simulink model "RobotX_ss_acousticsSKIP_dock_odoa_refer_model1021"  (R2014a)
settings: Solver=FixedStepDiscrete  StartTime=0.0  StopTime=inf  FixedStep=.25  RelTol=1e-3
undefined symbols (not defined in the file): Com1, Com2, Com3, Com4, DiscIntNeverNeededParam, standard
libraries: xpcseriallib x42, slrtlib x8, simulink x7, speedgoatlib x2, speedgoatlib_IO102 x1
(part 4 of 18)

== matlab function RobotX_ss_acousticsSKIP_dock_odoa_refer_model1021/Main FSM/ODOA/SLAM1/SLAM enabled/slammed ==
  data: mpa output; lm_data input; pre_part_positions input; part_positions output; positionboat input
%% SLAM by Chidananda Matada Shivananda
%  Copyright 2010 Randolph Voorhies

%  Edited 2014 Nick DiLeo - Modifications for unknown data association
%  and multiple measurements in a single timestep
    
%  Edited 2014 Chidananda Matada Shivananda - Simulink compatability, New
%  clustering technique added

%  This program is free software: you can redistribute it and/or modify
%  it under the terms of the GNU General Public License as published by
%  the Free Software Foundation, either version 3 of the License, or
%  (at your option) any later version.
%
%  This program is distributed in the hope that it will be useful,
%  but WITHOUT ANY WARRANTY; without even the implied warranty of
%  MERCHANTABILITY or FITNESS FOR A PARTICULAR PURPOSE.  See the
%  GNU General Public License for more details.
%
%  You should have received a copy of the GNU General Public License
%  along with this program.  If not, see <http://www.gnu.org/licenses/>.

function [mpa,part_positions]   = slammed(lm_data,pre_part_positions,positionboat)

%% General comments

% the angles in radians
% the ditance in m

%% Initialisations.

persistent particles avg_robot;
num_particles = 50;

% the limits
max_read_distance = 10;
min_read_distance = 5;
min_read_angle = -67.5*pi/180; %radians- maximum read angle
max_read_angle = 67.5*pi/180;

% The initial starting position of the robot Use UTM coordinates from GPS
avg_robot_position = [0;0;0];% x y rotation

% The Gaussian variance of the movement commands
% Approximating there are only two drives
% movement_variance = [.1;.1];   % Left drive Right_drive
% M = [movement_variance(1), 0.0;
%      0.0, movement_variance(2)];
measurement_variance = [0.01; 0.01];   % Distance Angle
R = [measurement_variance(1), 0.0;
    0.0, measurement_variance(2)];

default_importance=0.001;

if isempty(particles)
    %  Particles
    %             w[1]
    %             position[1,3]
    %             num_landmarks[300] this is to keep history
    
    %             lm_weight[2,15]based on number of landmarks
    %             landmarks[15]
    %                         position[2,1]
    %                         E[2,2]
    %                         counter[1]
    particles=repmat(struct('w',1.0/num_particles,'position',avg_robot_position,'num_landmarks',zeros(1,2),'lm_weight',repmat(1.0/num_particles,10,15),'landmarks',repmat(struct('pos',zeros(1,2),'E',zeros(2,2),'counter',0),1,15)),1,50);
    avg_robot_position = average_pos(particles,num_particles);
end

if isempty(avg_robot)
    avg_robot=avg_robot_position;
end

avg_robot_position=avg_robot;

%% Upload the moved data onto the particles
for shiva9=1:50
    particles(shiva9).position(1)= pre_part_positions(3*(shiva9-1)+1);
    particles(shiva9).position(2)= pre_part_positions(3*(shiva9-1)+1)*(pi/180);
    particles(shiva9).position(3)= pre_part_positions(3*(shiva9-1)+1);
end

%% Try to take a reading from each landmark and calculate the Jacobian
doResample = false;
% The input got from landmarks
[~,cols]=find(lm_data ~= 0);
if (isempty(cols)==0)% if the cols is not empty
    doResample=true; %if there is new measurement, then resample particles
end

if (doResample==true)
%     [r,~]=size(cols);
    [~,r]=size(cols);
    shiva=1;
    G=zeros(2,2,ceil(r/2));
    z_real=zeros(2,ceil(r/2));
    read_distance=zeros(ceil(r/2));
    read_angle=zeros(ceil(r/2));
    
    for lIdx = 1:2:r %amount of visible landmarks
        real_landmark = [lm_data(cols(lIdx+1)),lm_data(cols(lIdx))];
        % Take a real (noisy) measurement from the robot to the landmark
        %         [z_real(:,lIdx), G(:,:,lIdx)] = getRealMeasurement(avg_robot_position, real_landmark, [0 0]);
        %         function [z, H] = getRealMeasurement(pos, landmark_pos, observation_variance)
        
        landmark_angle=real_landmark(1);
        landmark_distance=real_landmark(2);
        % Compute the Jacobian of this measurement function
        q = landmark_distance^2.0;
        G(:,:,shiva) = [-(real_landmark(1) - avg_robot_position(1))/sqrt(q), -(real_landmark(2) - avg_robot_position(2))/sqrt(q);
            (real_landmark(2) - avg_robot_position(2))/q,       -(real_landmark(1) - avg_robot_position(1))/q];
        
        z_real(:,shiva) = [landmark_distance; landmark_angle];
        read_distance(shiva) = z_real(1,shiva);
        read_angle(shiva)    = z_real(2,shiva);
        shiva=shiva+1;
    end
    %     shiva=1;
    
    for pIdx = 1:num_particles
        %     particles(pIdx).lm_weight=[];
        %     clear z_p H Q
        %         coder.varsize('H', [2,2,16],[0 0 1]);
        num_landmarks=particles(pIdx).num_landmarks(1);
        assert(num_landmarks<20);
        H=zeros(2,2,num_landmarks);
        %         coder.varsize('z_p', [2 1 16]);
        z_p=zeros(2,1,num_landmarks);
        Q=zeros(2,2,num_landmarks);
        for j=1:particles(pIdx).num_landmarks(1)
            %             [z_p(:,j), H(:,:,j)] = getMeasurement(particles(pIdx).position, particles(pIdx).landmarks(j).pos, [0 0]);
            %             function [z, H] = getRealMeasurement(pos, landmark_pos, observation_variance)
            landmark_angle=particles(pIdx).landmarks(j).pos(1);
            landmark_distance=particles(pIdx).landmarks(j).pos(2);
            
            % Compute the Jacobian of this measurement function
            q = landmark_distance^2.0;
            %   H = [-(landmark_pos(1) - pos(1))/sqrt(q), -(landmark_pos(2) - pos(2))/sqrt(q), 0.0;
            %         (landmark_pos(2) - pos(2))/q,       -(landmark_pos(1) - pos(1))/q,      -1.0;
            %         0.0,                                0.0,                               1.0];
            
            H(:,:,j) = [-(particles(pIdx).landmarks(j).pos(1) - particles(pIdx).position(1))/sqrt(q), -(particles(pIdx).landmarks(j).pos(2) - particles(pIdx).position(2))/sqrt(q);
                (particles(pIdx).landmarks(j).pos(2) - particles(pIdx).position(2))/q,       -(particles(pIdx).landmarks(j).pos(1) - particles(pIdx).position(1))/q];
            
            
            z_p(:,j) = [landmark_distance;
                landmark_angle];
            
            for measured_lm=1:size(z_real,2)
                residual = z_real(:,measured_lm) - z_p(:,j);
                Q(:,:,j) = H(:,:,j)' * particles(pIdx).landmarks(j).E * H(:,:,j) + R;
                particles(pIdx).lm_weight(measured_lm,j) = particles(pIdx).w * norm(2*pi*Q(:,:,j)).^(-1/2)*exp(-1/2*(residual'/Q(:,:,j)*residual));
            end
        end
        
        particles(pIdx).num_landmarks(2)=particles(pIdx).num_landmarks(1);
        num_landmarks2=particles(pIdx).num_landmarks(2);
        assert(num_landmarks2<20);
        
        %           clear c_hat
        %         clear cost_table data_associate_mat data_associate_vect
        %%%%%%%%%%%%%%%%%%%%%%%%%%%%%%%%%%%%%%%%%%%%%%%%%%%%%%%%%%%%%%%%%%%%%%%%%%%%%%%%%%%%%%%%%%%%%%%%%%%%%%%%%%%%%%%%%%%%%%%%%%%%%%%%%%%%%%%%%%%%%
        cost_table=zeros(size(z_real,2),num_landmarks+size(z_real,2));
        %         cost_table=zeros(size(z_real,2),num_landmarks);
        
        if (num_landmarks~=0)
            cost_table(1:size(z_real,2),1:particles(pIdx).num_landmarks(1))=particles(pIdx).lm_weight(1:size(z_real,2),1:particles(pIdx).num_landmarks(1));
        end
        cost_table(1:size(z_real,2),particles(pIdx).num_landmarks(1)+1:particles(pIdx).num_landmarks(1)+size(z_real,2)) =default_importance*eye(size(z_real,2));
        
        particles(pIdx).w=max(max(cost_table,[],1),[],2);
        [~, idx_hold]=max(cost_table,[],1); %this is the max correseponding for each measurement
        for i=1:size(cost_table,2)
            idx_zero=setdiff(1:size(cost_table,1),idx_hold(i));
            cost_table(idx_zero,i)=0;
        end
        
        cost_table1=cost_table;
        for shiva14=1:size(cost_table,2)
            cost_table(:,shiva14)=cost_table1(:,size(cost_table,2)-shiva14+1);
        end
        
        
        new_landmarks=0;
        for measured_lm=1:size(z_real,2)
            [~, IDX] = max(cost_table(measured_lm,:));
            if IDX > particles(pIdx).num_landmarks(1)
                new_landmarks=new_landmarks+1;
            end
        end
        
        
        assert(new_landmarks<20);
        data_associate_mat=zeros(size(z_real,2),new_landmarks+num_landmarks2);
        
        for measured_lm=1:size(z_real,2)
            [~, IDX] = max(cost_table(measured_lm,:));
            if IDX > particles(pIdx).num_landmarks(1)
                %we haven't seen this landmark before
                %                 if particles(pIdx).num_landmarks(2)>14
                %                     break;
                %                 end
                particles(pIdx).num_landmarks(2)=particles(pIdx).num_landmarks(2)+1; %add new landmark
                data_associate_mat(measured_lm,particles(pIdx).num_landmarks(2))=measured_lm; %set correspondance b/t measurement and feature j
            else
                %we've already seen this landmark
                %           [val idx]=max(particles(pIdx).lm_weight(measured_lm,:));
                data_associate_mat(measured_lm,IDX)=measured_lm; %measurement is a known feature
            end
            
        end
        
        num_landmarks2=particles(pIdx).num_landmarks(2);
        assert(num_landmarks2<20);
        Hn=zeros(2,2,num_landmarks2);
        t=size(H);
        for i=1:t(3)
            Hn(:,:,i)=H(:,:,i);
        end
        
        %         H=zeros(2,2,num_landmarks2);
        H=Hn;
        
        data_associate_vect=max(data_associate_mat,[],1); %vector that contains measurement correspondance to landmarks
        i=1;
        feature_to_delete=zeros(num_landmarks2);
        for j=1:particles(pIdx).num_landmarks(2) %length(data_associate_vect)
            if (data_associate_vect(j)>0 && j>particles(pIdx).num_landmarks(1))
                % If we have never seen this landmark, then we need to initialize it.
                % We'll just use whatever first reading we recieved.
                particles(pIdx).landmarks(j).pos = [particles(pIdx).position(1) + ...
                    sin(read_angle(data_associate_vect(j))+particles(pIdx).position(3))*read_distance(data_associate_vect(j));...
                    particles(pIdx).position(2) + cos(read_angle(data_associate_vect(j))+particles(pIdx).position(3))*read_distance(data_associate_vect(j))]';
                % Initialize the landmark position covariance
                H(:,:,j)=G(:,:,data_associate_vect(j));
                particles(pIdx).landmarks(j).E = inv(G(:,:,data_associate_vect(j)))' * R * inv(G(:,:,data_associate_vect(j)));
                particles(pIdx).landmarks(j).counter=1; %initialize counter
            elseif (data_associate_vect(j)>0 && j<=particles(pIdx).num_landmarks(1))
                %we've seen this landmark before
                K = particles(pIdx).landmarks(j).E * H(:,:,j) / Q(:,:,j);
                % Mix the ideal reading, and our actual reading using the Kalman gain, and use the result
                % to predict a new landmark position
                particles(pIdx).landmarks(j).pos = particles(pIdx).landmarks(j).pos + (K*(z_real(:,data_associate_vect(j))-z_p(:,j)))';
                % Update the covariance of this landmark
                particles(pIdx).landmarks(j).E = (eye(size(H(:,:,j))) - K*H(:,:,j)')*particles(pIdx).landmarks(j).E;
                particles(pIdx).landmarks(j).counter=particles(pIdx).landmarks(j).counter+1; %increment counter
            else
                % We are leaving these unchanged.  These are commented
                % out, but this is what is actually happening in alg.
                % particles(pIdx).landmarks(j).pos = particles(pIdx).landmarks(j).pos;
                % particles(pIdx).landmarks(j).E=particles(pIdx).landmarks(j).E;
                dist_to_landmark=norm([particles(pIdx).landmarks(j).pos(1)-particles(pIdx).position(1) particles(pIdx).landmarks(j).pos(2)-particles(pIdx).position(2)]);
                ang_to_landmark=atan2((particles(pIdx).landmarks(j).pos(1) - particles(pIdx).position(1)),...
                    (particles(pIdx).landmarks(j).pos(2) - particles(pIdx).position(2)))-particles(pIdx).position(3);
                if (dist_to_landmark > max_read_distance ||dist_to_landmark < min_read_distance || ang_to_landmark > max_read_angle || ang_to_landmark < min_read_angle)
                    %counter(pIdx,j)=counter(pIdx,j) %don't change counter
                else
                    particles(pIdx).landmarks(j).counter=particles(pIdx).landmarks(j).counter-1; %decrement counter
                    if particles(pIdx).landmarks(j).counter<0
                        feature_to_delete(i)=j; %we're going to delete all these features at the end of the loop
                        i=i+1;
                    end
                end
                %
            end %if
        end %end j
        %     'pos',zeros(1,2),'E',zeros(2,2),'counter',0
        if~(isempty(nonzeros(feature_to_delete)))
            tobe_del=nonzeros(feature_to_delete);
            for shiva4=1:length(feature_to_delete)
                particles(pIdx).landmarks(tobe_del(shiva4)).pos=zeros(1,2);
                particles(pIdx).landmarks(tobe_del(shiva4)).E=zeros(2,2);
                particles(pIdx).landmarks(tobe_del(shiva4)).counter=0;
            end
            particles(pIdx).num_landmarks(2)= particles(pIdx).num_landmarks(2)-length(tobe_del);
        end
        
        particles(pIdx).num_landmarks(1)=particles(pIdx).num_landmarks(2);
        
    end %pIdx
    
    particles=resample(particles) ;
    
    
    
end% if (doResample==true)


%% Clustering
landmarks_positions=zeros(15*50,2);
row_counter=0;
for pIdx=1:num_particles
    for j=1:15 %this should be index timestep when in full script
        row_counter=row_counter+1;
        landmarks_positions(row_counter,:)=particles(pIdx).landmarks(j).pos(1:2)';
    end
end

[mpa,]=cluster(landmarks_positions,lm_data,positionboat);
max(landmarks_positions),max(mpa)
% 
% mpadi=mpa(:,1);
% mpaan=((mpa(:,2)));


%% new data prediction

%     lm_data_ind=lm_data(:)~=0;
%     lm_data_ind(1)=0;
%     lm_data1=lm_data(lm_data_ind);
%     
%     for j=(length(lm_data)/2)+1:(length(lm_data))
%         if lm_data(j)<91
%             lm_data(j)=psi(i)+lm_data(j);
%         else
%             lm_data(j)=psi(i)+lm_data(j)-360;
%         end
%     end
%     
%     if length(lm_data~=0)
%         x1=x(i)+(lm_data(1:length(lm_data)/2)/100).*sind(lm_data((length(lm_data)/2)+1:length(lm_data)));
%         y1=y(i)+(lm_data(1:length(lm_data)/2)/100).*cosd(lm_data((length(lm_data)/2)+1:length(lm_data)));
%     end

% landmarks_positions
% mpa1
% mpa=mpa1;




%% Final changes to be persistent
avg_robot=avg_robot_position;
part_positions=zeros(150,1);

for shiva9=1:3:150
    part_positions(shiva9)=particles(ceil(shiva9/3)).position(1);
    part_positions(shiva9+1)=(particles(ceil(shiva9/3)).position(2))*(180/pi);
    part_positions(shiva9+2)=particles(ceil(shiva9/3)).position(3);
end

%% Display and output

end %function [y,y1]  = slammed(imu_data,lm_data)

function [map,mapconv]= cluster(data,lm_add,positionboat)

n=size(data,1);
clusters=ones(n,1);
hubs=zeros(n,1);
hubs(1,1)=1;
dif=zeros(n,2);
% clustersort=zeros(n,3);
for i = 1:n
    dif(i,:)= data(clusters(i),:) - data(i,:);
end

dist =sum((dif.*dif),2);
counter =1;             %Keeps track of number of the present number of hubs
continue12 = 1;   % 1=true 0=false indicates whether to continue forming new
% rearr_lm(:,1)=lm_add(1:2:24)+rand(1);

while continue12
    counter = counter + 1;    % adding new hub
    if counter>750
        break;
    end
    [~,i]=max(dist);        %m= maximum value in the distance array
    %i is the location of the maximum value in the
    % array
    hubs(counter)=i;        %assigns index to new hub
    temp = i*ones(n,1);
    dif1=zeros(n,2);
    for i23 = 1:n
        dif1(i23,:)= data(temp(i23),:) - data(i23,:);
    end
    newdist =sum((dif1.*dif1),2);
    for r=1:n
        if newdist(r) < dist(r)
            dist(r)=newdist(r);
            clusters(r)=i;
        end     %end for if
    end
    maxdist=max(dist);      %returns distance of point farthest from its hub
    continue12 = farout(counter,hubs,data,maxdist); %Checks the stop condition
end

clustersort=[data,clusters];
clustersort=sortrows(clustersort,3);
map=zeros(12,2);
temp=zeros(12,1);
temp(1,1)=clustersort(1,3);
shiva12=1;
for i=1:n
    if sum(temp==clustersort(i,3)) == 0
        shiva12=shiva12+1;
        if shiva12>12
            break
        end
        temp(shiva12)=clustersort(i,3);
    end
end
for shiva13=1:12
    clusterIdx = clustersort(:,3)==temp(shiva13);
    map(shiva13,:)=[sum(clustersort(clusterIdx,1)),sum(clustersort(clusterIdx,2))]/(sum(clusterIdx)*50);
end
map(isnan(map))=0;

x=positionboat(1);
y=positionboat(2);
psi=positionboat(3);
for shiva17=1:2:23
    lm_add(shiva17+1)=lm_add(shiva17+1)*(180/pi);
    if lm_add(shiva17+1)<91
        lm_add(shiva17+1)=psi+lm_add(shiva17+1);
    else
        lm_add(shiva17+1)=psi+lm_add(shiva17+1)-360;
    end
end

shiva18=1;
mapconv=zeros(12,2);
for shiva17=1:2:23
    if (lm_add(shiva17)~=0 && lm_add(shiva17+1)~=0)
        mapconv(shiva18,1)=x+(lm_add(shiva17)*sind(lm_add(shiva17+1)));
        mapconv(shiva18,2)=y+(lm_add(shiva17)*cosd(lm_add(shiva17+1)));
        shiva18=shiva18+1;
    end
end

% map=map.*0.02;
for shiva19=1:12
   if (map(shiva19,1)<1000 && map(shiva19,1)~=0)
       map(shiva19,1)=map(shiva19,1)+4216.58; 
   end
   if (map(shiva19,2)<500 && map(shiva19,1)~=0)
       map(shiva19,2)=map(shiva19,2)+964; 
   end
end
% map(:,1)=map(:,1)+4216.58;
% map(:,2)=map(:,2)+964;
% map=map;
% map=map;
end

function continue1 = farout(counter1,hubs1,data1,maxdist1)

%FAROUT continue = farout(counter,hubs,data,maxdist)
%       Calculates stop condition.  Stops if the point farthest from its
%       hub is within the average distance value.

index1 = 0;
n=size(data1,1);
dif=zeros(n,2);
for i1 = 1:(counter1-1)
    for j = i1+1 : counter1
        index1 = index1 + 1;
        if index1>750
            break
        end
        dif(index1,:)=data1(hubs1(i1),:) - data1(hubs1(j),:);
    end
end

dist=sqrt(sum((dif.*dif),2));
average_dist = sum(dist)/(2*index1);
if (sqrt(maxdist1) < (average_dist/100000))
    continue1 = 0;
else continue1 =1;
end
end                             % end for farout

function avg_robot_position = average_pos(particles,num_particles)
xsiva=0;
ysiva=0;
rotasiva=0;

for siva=1:num_particles
    xsiva=xsiva+particles(siva).position(1);
    ysiva=ysiva+particles(siva).position(2);
    rotasiva=rotasiva+particles(siva).position(3);
end

avg_robot_position = [xsiva/num_particles; ysiva/num_particles; rotasiva/num_particles];

end

function [newParticles] = resample(oldParticles)
% Resample a group of particles such that those with higher weights have a
% higher chance of being replicated, and those with low weights have a high
% chance of disappearing
num_particles=50;
avg_robot_position = [0;0;0];% x y rotation
newParticles=repmat(struct('w',1.0/num_particles,'position',avg_robot_position,'num_landmarks',zeros(1,2),'lm_weight',repmat(1.0/num_particles,10,15),'landmarks',repmat(struct('pos',zeros(1,2),'E',zeros(2,2),'counter',0),1,15)),1,50);

weightSum = 0;
for i=1:length(oldParticles)
    weightSum = weightSum + oldParticles(i).w;
end
for i=1:length(oldParticles)
    oldParticles(i).w = oldParticles(i).w/weightSum;
end
M = length(oldParticles);
%   newParticles = [];
r = rand / M;
c = oldParticles(1).w;
i = 1;
shiva6=1;
assert(shiva6<51);
for m=1:M
    U = r + (m-1) * M^(-1);
    while U > c
        i = i+1;
        c = c+oldParticles(i).w;
    end
    newParticles(shiva6) = oldParticles(i);
    shiva6=shiva6+1;
end
for i=1:length(newParticles)
    newParticles(i).w = 1.0/length(newParticles);
end
end

== system RobotX_ss_acousticsSKIP_dock_odoa_refer_model1021/Main FSM/ODOA/GPS Move ==
  Sensors : Inport
  Enable : EnablePort
  Bus Selector : BusSelector  OutputSignals=Sensors.Navigation Message.Pose.X,Sensors.Navigation Message.Pose.Y,Sensors.Navigation Message.Pose.Psi,Sensors.Navigation Message.Velocity.u,Sensors
  CalcTimes : MATLAB Function  TreatAsAtomicUnit=on
  Data Store Read2 : DataStoreRead  DataStoreName=odoaGPS
  Data Store Read4 : DataStoreRead  DataStoreName=NED_origin
  Data Store Read5 : DataStoreRead  DataStoreName=ODOAentry
  GPSMove : MATLAB Function  TreatAsAtomicUnit=on
  LLA to NED1 : MATLAB Function  TreatAsAtomicUnit=on
  Output Reassign : Subsystem
  Outputs : Outport
  Finished : Outport  Port=2
  wires:
  GPSMove/3(pts) -> CalcTimes/1(pts)
  Sensors/1 -> Bus Selector/1
  Bus Selector/1 -> GPSMove/2(X)  "<X>"
  Bus Selector/2 -> GPSMove/3(Y)  "<Y>"
  Bus Selector/3 -> GPSMove/4(Psi)  "<Psi>"
  Bus Selector/4 -> CalcTimes/2(u)  "<u>"
  GPSMove/1(Finished) -> Finished/1
  Output Reassign/1(Outputs) -> Outputs/1
  CalcTimes/1(Data) -> Output Reassign/2(Data)
  GPSMove/2(valid) -> Output Reassign/1(Vaild)
  LLA to NED1/1(NEDout) -> GPSMove/1(GoalNED)
  Data Store Read2/1 -> LLA to NED1/2(LLAs)
  Data Store Read4/1 -> LLA to NED1/3(NED_origin)
  Data Store Read5/1 -> LLA to NED1/1(enterGate)
  Bus Selector/5 -> Output Reassign/3(Sensors)  "<Sensors>"

== system RobotX_ss_acousticsSKIP_dock_odoa_refer_model1021/Main FSM/ODOA/Path ==
  note: Through Gate
  Sensors : Inport
  Enable : EnablePort  ShowOutputPort=on
  A Star (Held Length) : MATLAB Function  TreatAsAtomicUnit=on
  Bus Selector : BusSelector  OutputSignals=Sensors.Navigation Message.Pose.X,Sensors.Navigation Message.Pose.Y,Sensors.Navigation Message.Pose.Psi,map,Sensors
  Bus Selector1 : BusSelector  OutputSignals=Navigation Message.Velocity.u
  Calculate Times : MATLAB Function  TreatAsAtomicUnit=on
  Data Store Read : DataStoreRead  DataStoreName=odoaGPS
  Data Store Read1 : DataStoreRead  DataStoreName=NED_origin
  Data Store Read2 : DataStoreRead  DataStoreName=ODOAexit
  Discrete-Time Integrator : DiscreteIntegrator  SampleTime=-1  ICPrevOutput=DiscIntNeverNeededParam  ICPrevScaledInput=DiscIntNeverNeededParam
  LLA to NED : MATLAB Function  TreatAsAtomicUnit=on
  Map Grid (Held Length) : MATLAB Function  TreatAsAtomicUnit=on
  Output Reassign : Subsystem
  Path To Trajectory : MATLAB Function  TreatAsAtomicUnit=on
  Outputs : Outport
  Finished : Outport  Port=2
  wires:
  Output Reassign/1(Outputs) -> Outputs/1
  Enable/1 -> Discrete-Time Integrator/1
  Map Grid (Held Length)/1(relPose) -> A Star (Held Length)/1(relPose), Path To Trajectory/2(relPose)
  Map Grid (Held Length)/2(obGrid) -> A Star (Held Length)/2(obGrid)
  Map Grid (Held Length)/3(targetPt) -> A Star (Held Length)/3(targetPt)
  A Star (Held Length)/1(Path) -> Path To Trajectory/3(Path)
  Map Grid (Held Length)/4(nodes) -> Path To Trajectory/4(nodes)
  Data Store Read2/1 -> Map Grid (Held Length)/1(exitGate)
  LLA to NED/1(NEDout) -> Map Grid (Held Length)/2(NEDcorners)
  Bus Selector/2 -> Map Grid (Held Length)/4(Y)  "<Y>"
  Bus Selector/3 -> Map Grid (Held Length)/5(Psi)  "<Psi>"
  Bus Selector/4 -> Map Grid (Held Length)/6(NEDlandmarks)  "<map>"
  Bus Selector/1 -> Map Grid (Held Length)/3(X)  "<X>"
  Path To Trajectory/3(trajectory) -> Calculate Times/1(pts)
  Bus Selector1/1 -> Calculate Times/2(u)  "<u>"
  Path To Trajectory/2(valid) -> Output Reassign/1(Vaild)
  Calculate Times/1(Data) -> Output Reassign/2(Data)
  Sensors/1 -> Bus Selector/1
  Discrete-Time Integrator/1 -> Path To Trajectory/1(time)
  Path To Trajectory/1(finished) -> Finished/1
  Data Store Read/1 -> LLA to NED/1(LLAs)
  Data Store Read1/1 -> LLA to NED/2(NED_origin)
  Bus Selector/5 -> Output Reassign/3(Sensors), Bus Selector1/1  "<Sensors>"

== system RobotX_ss_acousticsSKIP_dock_odoa_refer_model1021/Main FSM/ODOA/SLAM1 ==
  note: And conversions back to degrees needed for part_positions when it goes to input selection
  note: Conversion of angles to radians needed at SLAM pre_past_positions
  note: m and degrees
  note: m and degrees
  note: the models need in m and degrees
  note: LIDAR data in cm and deg
  note: Navigation m and degrees
  note: SLAM m and radians
  Sensors : Inport
  Any Landmark Change : MATLAB Function  TreatAsAtomicUnit=on
  Any State Change : MATLAB Function  TreatAsAtomicUnit=on
  Bus Selector : BusSelector  OutputSignals=Navigation Message,Lidar Data Input
  Bus Selector1 : BusSelector  OutputSignals=Landmarks.Distances,Landmarks.Angles
  Bus Selector2 : BusSelector  OutputSignals=Pose
  Detect Change : simulink/Logic and Bit Operations/Detect Change  vinit=0  InputProcessing=Inherited  OutDataTypeStr=boolean
  Detect Change1 : simulink/Logic and Bit Operations/Detect Change  vinit=0  InputProcessing=Inherited  OutDataTypeStr=boolean
  Landmark Organizer : MATLAB Function  TreatAsAtomicUnit=on
  Models for prediction : Subsystem
  SLAM enabled : Subsystem  TreatAsAtomicUnit=on
  inputselection : Subsystem
  map : Outport
  wires:
  Sensors/1 -> Bus Selector/1
  Bus Selector/1 -> Models for prediction/1(Nav Messages), Bus Selector2/1, Detect Change/1  "<Navigation Message>"
  Bus Selector/2 -> Bus Selector1/1  "<Lidar Data Input>"
  Bus Selector1/1 -> Landmark Organizer/1(Distances)  "<Distances>"
  Bus Selector1/2 -> Landmark Organizer/2(Angles)  "<Angles>"
  Landmark Organizer/1(lm_data) -> SLAM enabled/2(lm_data), Detect Change1/1
  Detect Change/1 -> Any State Change/1(u)
  Detect Change1/1 -> Any Landmark Change/1(u)
  Any Landmark Change/1(y) -> SLAM enabled/Enable, inputselection/3(Landmarkchange)
  Bus Selector2/1 -> inputselection/2(xypsi), SLAM enabled/3(positionboat)  "<Pose>"
  Any State Change/1(y) -> inputselection/1(controlchange)
  SLAM enabled/2(part_positions) -> inputselection/4(part_positions)
  inputselection/1(last particle positions) -> Models for prediction/2(xypsi150)
  Models for prediction/1(xypsioutput) -> inputselection/5(xypsi150), SLAM enabled/1(pre_past_positions)
  SLAM enabled/1(mpa) -> map/1  "map"

== system RobotX_ss_acousticsSKIP_dock_odoa_refer_model1021/Main FSM/RCHold/Direct Control ==
  Sensors : Inport
  Acoustic Active : Constant  Value=0
  Bus Creator2 : BusCreator  Inputs=3
  Bus Creator3 : BusCreator  Inputs=3
  Bus Creator4 : BusCreator  Inputs=2
  Constant : Constant
  Constant1 : Constant  Value=2
  Constant2 : Constant  Value=zeros(24,1)
  Lidar Mode : Constant  Value=3
  Outputs : Outport
  wires:
  Sensors/1 -> Bus Creator4/2  "Sensors"
  Bus Creator4/1 -> Outputs/1  "Output Signals"
  Bus Creator2/1 -> Bus Creator3/1  "Navigation Outputs"
  Acoustic Active/1 -> Bus Creator3/2  "Acoustic Active"
  Lidar Mode/1 -> Bus Creator3/3  "Lidar Mode"
  Bus Creator3/1 -> Bus Creator4/1  "Outputs"
  Constant/1 -> Bus Creator2/1  "Valid"
  Constant1/1 -> Bus Creator2/2  "Control Mode"
  Constant2/1 -> Bus Creator2/3  "Data"

== system RobotX_ss_acousticsSKIP_dock_odoa_refer_model1021/Main FSM/Start//Speedgate/Aim ==
  note: Signal
  Sensors : Inport
  Enable : EnablePort  ShowOutputPort=on
  Compare To Constant : simulink/Logic and Bit Operations/Compare To Constant  relop=>=  const=30  OutDataTypeStr=boolean
  Data Store Read : DataStoreRead  DataStoreName=ssHeldHeading
  Data Store Read1 : DataStoreRead  DataStoreName=ssGateGPS
  Data Store Read2 : DataStoreRead  DataStoreName=NED_origin
  Data Store Read3 : DataStoreRead  DataStoreName=Course
  Data Type Conversion : DataTypeConversion  OutDataTypeStr=double
  Discrete-Time Integrator : DiscreteIntegrator  SampleTime=-1  ICPrevOutput=DiscIntNeverNeededParam  ICPrevScaledInput=DiscIntNeverNeededParam
  LLA to NED : MATLAB Function  TreatAsAtomicUnit=on
  MATLAB Function : MATLAB Function  TreatAsAtomicUnit=on
  Output Heirarchy : Subsystem
  Outputs : Outport
  Finished : Outport  Port=2
  wires:
  Discrete-Time Integrator/1 -> Compare To Constant/1
  Enable/1 -> Discrete-Time Integrator/1
  Compare To Constant/1 -> Data Type Conversion/1
  Data Type Conversion/1 -> Finished/1
  Sensors/1 -> Output Heirarchy/2(Sensors)
  MATLAB Function/1(Data) -> Output Heirarchy/1(Data)
  Output Heirarchy/1(Outputs) -> Outputs/1
  Data Store Read/1 -> MATLAB Function/1(ssHeldHeading)
  LLA to NED/1(GoalNED) -> MATLAB Function/2(ssGateNED)
  Data Store Read1/1 -> LLA to NED/2(LLAs)
  Data Store Read2/1 -> LLA to NED/3(NED_origin)
  Data Store Read3/1 -> LLA to NED/1(Course)

== system RobotX_ss_acousticsSKIP_dock_odoa_refer_model1021/Main FSM/Start//Speedgate/Dead Reckon ==
  note: Through Gate
  Sensors : Inport
  Enable : EnablePort
  Bus Selector : BusSelector  OutputSignals=Navigation Message.Pose.X,Navigation Message.Pose.Y,Navigation Message.Velocity.u
  Calculate Times : MATLAB Function  TreatAsAtomicUnit=on
  Data Store Read : DataStoreRead  DataStoreName=ssHeldHeading
  Gate : MATLAB Function  TreatAsAtomicUnit=on
  Output Reassign : Subsystem
  Outputs : Outport
  Finished : Outport  Port=2
  wires:
  Output Reassign/1(Outputs) -> Outputs/1
  Gate/1(Finished) -> Finished/1
  Sensors/1 -> Output Reassign/3(Sensors), Bus Selector/1
  Bus Selector/2 -> Gate/3(Y)  "<Y>"
  Bus Selector/1 -> Gate/2(X)  "<X>"
  Bus Selector/3 -> Calculate Times/2(u)  "<u>"
  Gate/3(pts) -> Calculate Times/1(pts)
  Calculate Times/1(Data) -> Output Reassign/2(Data)
  Gate/2(Valid) -> Output Reassign/1(Vaild)
  Data Store Read/1 -> Gate/1(ssHeldHeading)

== system RobotX_ss_acousticsSKIP_dock_odoa_refer_model1021/Main FSM/Start//Speedgate/GPS Move ==
  Sensors : Inport
  Enable : EnablePort
  Bus Selector : BusSelector  OutputSignals=Navigation Message.Pose.X,Navigation Message.Pose.Y,Navigation Message.Pose.Psi,Navigation Message.Velocity.u
  CalcTimes : MATLAB Function  TreatAsAtomicUnit=on
  Data Store Read1 : DataStoreRead  DataStoreName=ssGateGPS
  Data Store Read2 : DataStoreRead  DataStoreName=NED_origin
  Data Store Read3 : DataStoreRead  DataStoreName=Course
  GPSMove : MATLAB Function  TreatAsAtomicUnit=on
  LLA to NED : MATLAB Function  TreatAsAtomicUnit=on
  Output Reassign : Subsystem
  Outputs : Outport
  Finished : Outport  Port=2
  wires:
  GPSMove/3(pts) -> CalcTimes/1(pts)
  Sensors/1 -> Output Reassign/3(Sensors), Bus Selector/1
  Bus Selector/1 -> GPSMove/2(X)  "<X>"
  Bus Selector/2 -> GPSMove/3(Y)  "<Y>"
  Bus Selector/3 -> GPSMove/4(Psi)  "<Psi>"
  Bus Selector/4 -> CalcTimes/2(u)  "<u>"
  GPSMove/1(Finished) -> Finished/1
  Output Reassign/1(Outputs) -> Outputs/1
  CalcTimes/1(Data) -> Output Reassign/2(Data)
  GPSMove/2(valid) -> Output Reassign/1(Vaild)
  LLA to NED/1(GoalNED) -> GPSMove/1(GoalNED)
  Data Store Read1/1 -> LLA to NED/2(LLAs)
  Data Store Read2/1 -> LLA to NED/3(NED_origin)
  Data Store Read3/1 -> LLA to NED/1(Course)

== system RobotX_ss_acousticsSKIP_dock_odoa_refer_model1021/Main FSM/Termination/Output Reassign ==
  Vaild : Inport
  Data : Inport  Port=2
  Sensors : Inport  Port=3
  Acoustic Active : Constant  Value=0
  Bus Creator2 : BusCreator  Inputs=3
  Bus Creator3 : BusCreator  Inputs=3
  Bus Creator5 : BusCreator  Inputs=2
  Constant3 : Constant  Value=0
  Lidar Mode : Constant  Value=0
  Outputs : Outport
  wires:
  Sensors/1 -> Bus Creator5/2  "Sensors"
  Bus Creator5/1 -> Outputs/1  "Output Signals"
  Vaild/1 -> Bus Creator2/1  "Valid"
  Constant3/1 -> Bus Creator2/2  "Control Mode"
  Data/1 -> Bus Creator2/3  "Data"
  Bus Creator2/1 -> Bus Creator3/1  "Navigation Outputs"
  Acoustic Active/1 -> Bus Creator3/2  "Acoustic Active"
  Lidar Mode/1 -> Bus Creator3/3  "Lidar Mode"
  Bus Creator3/1 -> Bus Creator5/1  "Outputs"

== system RobotX_ss_acousticsSKIP_dock_odoa_refer_model1021/Sensors/1020 Comms/ Raspberry Pi LCM (Acoustic) ==
  LCM Input : Inport
  ASCII Decode 6 : xpcseriallib/ASCII Decode   format=Deploy:%1u, Elapsed:%g, Bearing1:%g Bearing2:%g \r\n  nvars=4  vartypes={}
  Bus Creator : BusCreator  Inputs=2
  Bus Creator1 : BusCreator  Inputs=3
  FIFO ASCII read 1 : xpcseriallib/FIFO ASCII read   header={'Deploy:'}  term=[13 10]  hold=Zero output if no new data  enable=off  maxsize=1024  outputtype=8 bit uint null terminated  sampletime=-1
  LCM Output : Outport
  wires:
  LCM Input/1 -> FIFO ASCII read 1/1
  FIFO ASCII read 1/1 -> ASCII Decode 6/1
  ASCII Decode 6/3 -> Bus Creator/1  "Horizontal Bearing"
  ASCII Decode 6/4 -> Bus Creator/2  "Vertical Bearing"
  Bus Creator/1 -> Bus Creator1/3  "Bearings"
  ASCII Decode 6/2 -> Bus Creator1/2  "Elapsed Time"
  ASCII Decode 6/1 -> Bus Creator1/1  "Deployed"
  Bus Creator1/1 -> LCM Output/1  "Acoustic Message"

== system RobotX_ss_acousticsSKIP_dock_odoa_refer_model1021/Sensors/1020 Comms/ Raspberry Pi LCM (Navigation and Acoustics) ==
  LCM Input : Inport
  ASCII Decode 6 : xpcseriallib/ASCII Decode   format=P1:%f P2:%f P3:%f V1:%f V2:%f V3:%f E1:%f E2:%f E3:%f Pt1:%f Pt2:%f St1:%f St2:%f Start:%f Elapsed:%f RC:%d Deploy:%u, Elapsed:%g, Bearing1:%g Bearing2:%g \r\n  nvars=22  vartypes={}
  Bus Creator{,5..7} (4 alike) : BusCreator  Inputs=2
  Bus Creator{1..3,8} (4 alike) : BusCreator  Inputs=3
  Bus Creator4 : BusCreator  Inputs=9
  Data Type Conversion : DataTypeConversion  OutDataTypeStr=double
  FIFO ASCII read 1 : xpcseriallib/FIFO ASCII read   header={'P1:'}  term=[13 10]  hold=Zero output if no new data  enable=off  maxsize=2048  outputtype=8 bit uint null terminated  sampletime=-1
  Navigation LCM : Outport
  Acoustic LCM : Outport  Port=2
  wires:
  LCM Input/1 -> FIFO ASCII read 1/1
  FIFO ASCII read 1/1 -> ASCII Decode 6/1
  Bus Creator4/1 -> Navigation LCM/1  "Navigation Message"
  ASCII Decode 6/1 -> Bus Creator1/1  "X"
  ASCII Decode 6/2 -> Bus Creator1/2  "Y"
  ASCII Decode 6/3 -> Bus Creator1/3  "Psi"
  Bus Creator1/1 -> Bus Creator4/1  "Pose"
  ASCII Decode 6/4 -> Bus Creator2/1  "u"
  ASCII Decode 6/5 -> Bus Creator2/2  "v"
  Bus Creator2/1 -> Bus Creator4/2  "Velocity"
  ASCII Decode 6/7 -> Bus Creator3/1  "Roll"
  ASCII Decode 6/8 -> Bus Creator3/2  "Pitch"
  ASCII Decode 6/9 -> Bus Creator3/3  "Yaw"
  Bus Creator3/1 -> Bus Creator4/3  "Euler"
  Bus Creator5/1 -> Bus Creator4/5  "Port"
  Bus Creator6/1 -> Bus Creator4/6  "Stbd"
  ASCII Decode 6/14 -> Bus Creator6/1  "StThrust"
  ASCII Decode 6/15 -> Bus Creator6/2  "StAzimuth"
  ASCII Decode 6/12 -> Bus Creator5/1  "PtThrust"
  ASCII Decode 6/13 -> Bus Creator5/2  "PtAzimuth"
  ASCII Decode 6/16 -> Bus Creator4/7  "Start"
  ASCII Decode 6/17 -> Bus Creator4/8  "Elapsed"
  ASCII Decode 6/18 -> Data Type Conversion/1  "On/Off/RC/Auto"
  Data Type Conversion/1 -> Bus Creator4/9  "On/Off/RC/Auto"
  ASCII Decode 6/6 -> Bus Creator2/3  "r"
  ASCII Decode 6/10 -> Bus Creator7/1  "Lat"
  ASCII Decode 6/11 -> Bus Creator7/2  "Long"
  Bus Creator7/1 -> Bus Creator4/4  "GPS (LLA)"
  ASCII Decode 6/21 -> Bus Creator/1  "Horizontal Bearing"
  ASCII Decode 6/22 -> Bus Creator/2  "Vertical Bearing"
  Bus Creator/1 -> Bus Creator8/3  "Bearings"
  ASCII Decode 6/20 -> Bus Creator8/2  "Elapsed Time"
  ASCII Decode 6/19 -> Bus Creator8/1  "Deployed"
  Bus Creator8/1 -> Acoustic LCM/1  "Acoustic Message"

== system RobotX_ss_acousticsSKIP_dock_odoa_refer_model1021/Sensors/1020 Comms/ Raspberry Pi LCM (Navigation) ==
  LCM Input : Inport
  ASCII Decode 6 : xpcseriallib/ASCII Decode   format=P1:%f P2:%f P3:%f V1:%f V2:%f V3:%f E1:%f E2:%f E3:%f Lat:%f Long:%f Pt1:%f Pt2:%f St1:%f St2:%f Start:%f Elapsed:%f RC:%d Deploy:%u Elapsed:%f Bearing1:%f Bearing2:%f Range:%f X_Pos:%f Y_Pos:%f \r\n  nvars=25  vartypes={}
  Bus Creator1 : BusCreator  Inputs=3
  Bus Creator2 : BusCreator  Inputs=3
  Bus Creator3 : BusCreator  Inputs=3
  Bus Creator4 : BusCreator  Inputs=9
  Bus Creator5 : BusCreator  Inputs=2
  Bus Creator6 : BusCreator  Inputs=2
  Bus Creator7 : BusCreator  Inputs=2
  Bus Creator8 : BusCreator  Inputs=7
  Data Type Conversion : DataTypeConversion  OutDataTypeStr=double
  FIFO ASCII read 1 : xpcseriallib/FIFO ASCII read   header={'P1:'}  term=[13 10]  hold=Zero output if no new data  enable=off  maxsize=2000  outputtype=8 bit uint null terminated  sampletime=-1
  LCM Output : Outport
  Acou LCM : Outport  Port=2
  wires:
  LCM Input/1 -> FIFO ASCII read 1/1
  FIFO ASCII read 1/1 -> ASCII Decode 6/1
  Bus Creator4/1 -> LCM Output/1  "Navigation Message"
  ASCII Decode 6/1 -> Bus Creator1/1  "X"
  ASCII Decode 6/2 -> Bus Creator1/2  "Y"
  ASCII Decode 6/3 -> Bus Creator1/3  "Psi"
  Bus Creator1/1 -> Bus Creator4/1  "Pose"
  ASCII Decode 6/4 -> Bus Creator2/1  "u"
  ASCII Decode 6/5 -> Bus Creator2/2  "v"
  Bus Creator2/1 -> Bus Creator4/2  "Velocity"
  ASCII Decode 6/7 -> Bus Creator3/1  "Roll"
  ASCII Decode 6/8 -> Bus Creator3/2  "Pitch"
  ASCII Decode 6/9 -> Bus Creator3/3  "Yaw"
  Bus Creator3/1 -> Bus Creator4/3  "Euler"
  Bus Creator5/1 -> Bus Creator4/5  "Port"
  Bus Creator6/1 -> Bus Creator4/6  "Stbd"
  ASCII Decode 6/14 -> Bus Creator6/1  "StThrust"
  ASCII Decode 6/15 -> Bus Creator6/2  "StAzimuth"
  ASCII Decode 6/12 -> Bus Creator5/1  "PtThrust"
  ASCII Decode 6/13 -> Bus Creator5/2  "PtAzimuth"
  ASCII Decode 6/16 -> Bus Creator4/7  "Start"
  ASCII Decode 6/17 -> Bus Creator4/8  "Elapsed"
  ASCII Decode 6/18 -> Data Type Conversion/1  "On/Off/RC/Auto"
  Data Type Conversion/1 -> Bus Creator4/9  "On/Off/RC/Auto"
  ASCII Decode 6/6 -> Bus Creator2/3  "r"
  ASCII Decode 6/10 -> Bus Creator7/1  "Lat"
  ASCII Decode 6/11 -> Bus Creator7/2  "Long"
  Bus Creator7/1 -> Bus Creator4/4  "GPS (LLA)"
  ASCII Decode 6/19 -> Bus Creator8/1  "Deployed"
  ASCII Decode 6/20 -> Bus Creator8/2  "Elapsed Time"
  ASCII Decode 6/21 -> Bus Creator8/3  "Horizontal Bearing"
  ASCII Decode 6/22 -> Bus Creator8/4  "Vertical Bearing"
  ASCII Decode 6/23 -> Bus Creator8/5  "Range"
  ASCII Decode 6/24 -> Bus Creator8/6  "X Pos"
  ASCII Decode 6/25 -> Bus Creator8/7  "Y Pos"
  Bus Creator8/1 -> Acou LCM/1

== system RobotX_ss_acousticsSKIP_dock_odoa_refer_model1021/Sensors/1020 Comms/Acoustic LCM ==
  LCM Input : Inport
  Bus Creator : BusCreator  Inputs=2
  Bus Creator1 : BusCreator
  Bus Creator2 : BusCreator  Inputs=3
  Bus Selector : BusSelector  OutputSignals=Deployed,Elapsed Time,Horizontal Bearing,Vertical Bearing,Range,X Pos,Y Pos
  LCM Output : Outport
  wires:
  Bus Selector/3 -> Bus Creator/1  "<Horizontal Bearing>"
  Bus Selector/4 -> Bus Creator/2  "<Vertical Bearing>"
  Bus Creator/1 -> Bus Creator1/3  "Bearings"
  Bus Selector/2 -> Bus Creator1/2  "<Elapsed Time>"
  Bus Selector/1 -> Bus Creator1/1  "<Deployed>"
  Bus Creator1/1 -> LCM Output/1  "Acoustic Message"
  LCM Input/1 -> Bus Selector/1
  Bus Selector/5 -> Bus Creator2/1  "<Range>"
  Bus Selector/6 -> Bus Creator2/2  "<X Pos>"
  Bus Selector/7 -> Bus Creator2/3  "<Y Pos>"
  Bus Creator2/1 -> Bus Creator1/4  "Pose Estimate"

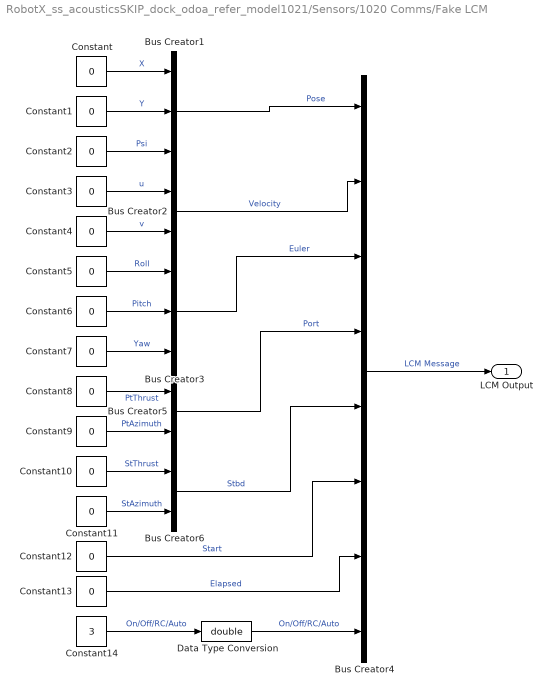
== system RobotX_ss_acousticsSKIP_dock_odoa_refer_model1021/Sensors/1020 Comms/Fake LCM ==
  Bus Creator1 : BusCreator  Inputs=3
  Bus Creator2 : BusCreator  Inputs=2
  Bus Creator3 : BusCreator  Inputs=3
  Bus Creator4 : BusCreator  Inputs=8
  Bus Creator5 : BusCreator  Inputs=2
  Bus Creator6 : BusCreator  Inputs=2
  Constant{,1..13} (14 alike) : Constant  Value=0
  Constant14 : Constant  Value=3
  Data Type Conversion : DataTypeConversion  OutDataTypeStr=double
  LCM Output : Outport
  wires:
  Bus Creator4/1 -> LCM Output/1  "LCM Message"
  Constant/1 -> Bus Creator1/1  "X"
  Constant1/1 -> Bus Creator1/2  "Y"
  Constant2/1 -> Bus Creator1/3  "Psi"
  Bus Creator1/1 -> Bus Creator4/1  "Pose"
  Constant3/1 -> Bus Creator2/1  "u"
  Constant4/1 -> Bus Creator2/2  "v"
  Bus Creator2/1 -> Bus Creator4/2  "Velocity"
  Constant5/1 -> Bus Creator3/1  "Roll"
  Constant6/1 -> Bus Creator3/2  "Pitch"
  Constant7/1 -> Bus Creator3/3  "Yaw"
  Bus Creator3/1 -> Bus Creator4/3  "Euler"
  Bus Creator5/1 -> Bus Creator4/4  "Port"
  Bus Creator6/1 -> Bus Creator4/5  "Stbd"
  Constant10/1 -> Bus Creator6/1  "StThrust"
  Constant11/1 -> Bus Creator6/2  "StAzimuth"
  Constant8/1 -> Bus Creator5/1  "PtThrust"
  Constant9/1 -> Bus Creator5/2  "PtAzimuth"
  Constant12/1 -> Bus Creator4/6  "Start"
  Constant13/1 -> Bus Creator4/7  "Elapsed"
  Constant14/1 -> Data Type Conversion/1  "On/Off/RC/Auto"
  Data Type Conversion/1 -> Bus Creator4/8  "On/Off/RC/Auto"

== system RobotX_ss_acousticsSKIP_dock_odoa_refer_model1021/Sensors/1020 Comms/LIDAR Panda ==
  LIDAR Panda In : Inport
  ASCII Decode 2 : xpcseriallib/ASCII Decode   format=A:%d B:%d C:%d E:%d F:%d G:%d H:%d I:%d J:%d K:%d L:%d M:%d N:%d O:%d P:%d Q:%d R:%d S:%d T:%d U:%d V:%d W:%d X:%d C1:%d C2:%d C3:%d C4:%d P1:%f P2:%f P3:%f P4:%f I1:%d I2:%d I3:%d I4:%d \r\n  nvars=36  vartypes={}
  Bus Creator1 : BusCreator  Inputs=2
  Bus Creator2 : BusCreator  Inputs=3
  Bus Creator3 : BusCreator  Inputs=2
  Data Type Conversion{,1..3} (4 alike) : DataTypeConversion  OutDataTypeStr=double
  "FIFO ASCII read " : xpcseriallib/FIFO ASCII read   header={'A:'}  term=[13 10]  hold=Zero output if no new data  enable=off  maxsize=1024  outputtype=8 bit uint null terminated  sampletime=-1
  Mux : Mux  Inputs=12
  Mux1 : Mux
  Mux2 : Mux  Inputs=12
  Mux3 : Mux
  Mux4 : Mux
  LIDAR Panda Out : Outport
  wires:
  LIDAR Panda In/1 -> "FIFO ASCII read "/1
  "FIFO ASCII read "/1 -> ASCII Decode 2/1
  ASCII Decode 2/3 -> Mux/3  "Distance"
  ASCII Decode 2/2 -> Mux/2  "Color ID"
  ASCII Decode 2/4 -> Mux/4  "Angle"
  ASCII Decode 2/1 -> Mux/1  "Probability"
  ASCII Decode 2/7 -> Mux/7
  ASCII Decode 2/10 -> Mux/10
  ASCII Decode 2/11 -> Mux/11
  ASCII Decode 2/6 -> Mux/6
  ASCII Decode 2/8 -> Mux/8
  ASCII Decode 2/9 -> Mux/9
  ASCII Decode 2/12 -> Mux/12
  ASCII Decode 2/5 -> Mux/5
  ASCII Decode 2/13 -> Mux2/1
  ASCII Decode 2/15 -> Mux2/3
  ASCII Decode 2/22 -> Mux2/10
  ASCII Decode 2/23 -> Mux2/11
  ASCII Decode 2/17 -> Mux2/5
  ASCII Decode 2/18 -> Mux2/6
  ASCII Decode 2/14 -> Mux2/2
  ASCII Decode 2/24 -> Mux2/12
  ASCII Decode 2/20 -> Mux2/8
  ASCII Decode 2/19 -> Mux2/7
  ASCII Decode 2/21 -> Mux2/9
  ASCII Decode 2/16 -> Mux2/4
  ASCII Decode 2/25 -> Mux1/1
  ASCII Decode 2/28 -> Mux1/4
  ASCII Decode 2/26 -> Mux1/2
  ASCII Decode 2/27 -> Mux1/3
  ASCII Decode 2/30 -> Mux3/2
  ASCII Decode 2/31 -> Mux3/3
  ASCII Decode 2/32 -> Mux3/4
  ASCII Decode 2/29 -> Mux3/1
  ASCII Decode 2/36 -> Mux4/4
  ASCII Decode 2/34 -> Mux4/2
  ASCII Decode 2/35 -> Mux4/3
  ASCII Decode 2/33 -> Mux4/1
  Mux/1 -> Data Type Conversion/1  "Distances"
  Mux2/1 -> Data Type Conversion1/1  "Angles"
  Mux1/1 -> Data Type Conversion2/1  "Color"
  Mux3/1 -> Bus Creator2/2  "Probability"
  Mux4/1 -> Data Type Conversion3/1  "idx"
  Bus Creator1/1 -> Bus Creator3/1  "Landmarks"
  Bus Creator2/1 -> Bus Creator3/2  "Color data"
  Bus Creator3/1 -> LIDAR Panda Out/1
  Data Type Conversion/1 -> Bus Creator1/1  "Distances"
  Data Type Conversion1/1 -> Bus Creator1/2  "Angles"
  Data Type Conversion2/1 -> Bus Creator2/1  "Color"
  Data Type Conversion3/1 -> Bus Creator2/3  "Color"

== system RobotX_ss_acousticsSKIP_dock_odoa_refer_model1021/Sensors/1020 Comms/Subsystem ==
  Bus Creator : BusCreator  Inputs=3
  Bus Creator1 : BusCreator  Inputs=2
  Bus Creator2 : BusCreator  Inputs=2
  Constant : Constant  Value=zeros(12,1)
  Constant1 : Constant  Value=zeros(12,1)
  Constant2 : Constant  Value=zeros(4,1)
  Constant3 : Constant  Value=zeros(4,1)
  Constant4 : Constant  Value=zeros(4,1)
  Fake Panda : Outport
  wires:
  Constant/1 -> Bus Creator1/1  "Distances"
  Constant1/1 -> Bus Creator1/2  "Angles"
  Constant2/1 -> Bus Creator/1  "Color"
  Constant3/1 -> Bus Creator/2  "Probability"
  Constant4/1 -> Bus Creator/3  "idx"
  Bus Creator1/1 -> Bus Creator2/1  "Landmarks"
  Bus Creator/1 -> Bus Creator2/2  "Color data"
  Bus Creator2/1 -> Fake Panda/1  "Lidar Data Input"

== system RobotX_ss_acousticsSKIP_dock_odoa_refer_model1021/Sensors/1020 Comms/data log ==
  Sensors signal : Inport
  Bus Selector3 : BusSelector  OutputSignals=Navigation Message,Lidar Data Input,Acoustic Message
  Bus to Vector : BusToVector
  Bus to Vector1 : BusToVector
  Bus to Vector2 : BusToVector
  Read : DataStoreRead  DataStoreName=PingPose
  Scope 1 : slrtlib/Displays and Logging/Scope   scopeno=3  scopetype=File  autostart=on  viewmode=Graphical redraw  formatstr='%15.6f'  grid=on  ylimits=[0,0]  nosamples=28800  noprepostsamples=0  interleave=1  triggermode=FreeRun  triggersignal=1  trigsignalfromport=off  triggerlevel=0.0  triggerslope=Either  triggerscope=1  triggersample=0  filename=LM1_<%%%>.dat  mode=Lazy  writesize=5120  autorestart=on  dynamicfilemode=on  maxwritefilesize=512*1024^2
  Scope 2 : slrtlib/Displays and Logging/Scope   scopeno=1  scopetype=File  autostart=on  viewmode=Graphical redraw  formatstr='%15.6f'  grid=on  ylimits=[0,0]  nosamples=28800  noprepostsamples=0  interleave=1  triggermode=FreeRun  triggersignal=1  trigsignalfromport=off  triggerlevel=0.0  triggerslope=Either  triggerscope=1  triggersample=0  filename=NAV1_<%%%>.dat  mode=Lazy  writesize=5120  autorestart=on  dynamicfilemode=on  maxwritefilesize=512*1024^2
  Scope 3 : slrtlib/Displays and Logging/Scope   scopeno=2  scopetype=File  autostart=on  viewmode=Graphical redraw  formatstr='%15.6f'  grid=on  ylimits=[0,0]  nosamples=28800  noprepostsamples=0  interleave=1  triggermode=FreeRun  triggersignal=1  trigsignalfromport=off  triggerlevel=0.0  triggerslope=Either  triggerscope=1  triggersample=0  filename=ACO1_<%%%>.dat  mode=Lazy  writesize=5120  autorestart=on  dynamicfilemode=on  maxwritefilesize=512*1024^2
  Scope 4 : slrtlib/Displays and Logging/Scope   scopeno=4  scopetype=File  autostart=on  viewmode=Graphical redraw  formatstr='%15.6f'  grid=on  ylimits=[0,0]  nosamples=28800  noprepostsamples=0  interleave=1  triggermode=FreeRun  triggersignal=1  trigsignalfromport=off  triggerlevel=0.0  triggerslope=Either  triggerscope=1  triggersample=0  filename=pPos_<%%%>.dat  mode=Lazy  writesize=5120  autorestart=on  dynamicfilemode=on  maxwritefilesize=512*1024^2
  wires:
  Sensors signal/1 -> Bus Selector3/1
  Bus to Vector/1 -> Scope 2/1
  Bus Selector3/1 -> Bus to Vector/1  "<Navigation Message>"
  Bus to Vector1/1 -> Scope 1/1
  Bus to Vector2/1 -> Scope 3/1
  Bus Selector3/3 -> Bus to Vector2/1  "<Acoustic Message>"
  Bus Selector3/2 -> Bus to Vector1/1  "<Lidar Data Input>"
  Read/1 -> Scope 4/1

== system RobotX_ss_acousticsSKIP_dock_odoa_refer_model1021/Sensors/1021 Comms/ Raspberry Pi LCM (Acoustic) ==
  LCM Input : Inport
  ASCII Decode 6 : xpcseriallib/ASCII Decode   format=Deploy:%1u, Elapsed:%g, Bearing1:%g Bearing2:%g \r\n  nvars=4  vartypes={}
  Bus Creator : BusCreator  Inputs=2
  Bus Creator1 : BusCreator  Inputs=3
  FIFO ASCII read 1 : xpcseriallib/FIFO ASCII read   header={'Deploy:'}  term=[13 10]  hold=Zero output if no new data  enable=off  maxsize=1024  outputtype=8 bit uint null terminated  sampletime=-1
  LCM Output : Outport
  wires:
  LCM Input/1 -> FIFO ASCII read 1/1
  FIFO ASCII read 1/1 -> ASCII Decode 6/1
  ASCII Decode 6/3 -> Bus Creator/1  "Horizontal Bearing"
  ASCII Decode 6/4 -> Bus Creator/2  "Vertical Bearing"
  Bus Creator/1 -> Bus Creator1/3  "Bearings"
  ASCII Decode 6/2 -> Bus Creator1/2  "Elapsed Time"
  ASCII Decode 6/1 -> Bus Creator1/1  "Deployed"
  Bus Creator1/1 -> LCM Output/1  "Acoustic Message"
